simulink model "mcecu_uds_on_fusion"  (Simulink 9.2)
settings: Solver=VariableStepAuto  StartTime=0.0  StopTime=10  RelTol=1e-3
undefined symbols (not defined in the file or in its folder): canChannel
libraries: canlib x3, canmsglib x3
settings Model: Creator=cordunoalbarran  LastModifiedBy=cordunoalbarran
settings DataIOCC: LimitDataPoints=off  SaveFormat=Dataset  SignalLoggingSaveFormat=Dataset
settings OptimizationCC: DefaultParameterBehavior=Inlined  EnhancedBackFolding=on  PassReuseOutputArgsThreshold=0  LifeSpan=auto  OptimizeBlockOrder=speed  DifferentSizesBufferReuse=on  OptimizationCustomize=off
settings DebuggingCC: UnderspecifiedInitializationDetection=Simplified  MergeDetectMultiDrivingBlocksExec=error  ParameterTunabilityLossMsg=error  FcnCallInpInsideContextMsg=error  StateNameClashWarn=none  SFUnexpectedBacktrackingDiag=error  SFNoUnconditionalDefaultTransitionDiag=error  SFExecutionAtInitializationDiag=warning
settings HardwareCC: ProdBitPerPointer=64  ProdBitPerSizeT=64  ProdBitPerPtrDiffT=64  ProdLargestAtomicFloat=Float  ProdIntDivRoundTo=Zero  ProdEndianess=LittleEndian  ProdWordSize=64  ProdHWDeviceType=Intel->x86-64 (Windows64)
settings ModelReferenceCC: PropagateSignalLabelsOutOfModel=on
settings SFSimCC: SimUseLocalCustomCode=on  MATLABDynamicMemAlloc=off
settings RTWCC: GenerateReport=on  RTWUseLocalCustomCode=on  LaunchReport=on
settings CodeAppCC: ForceParamTrailComments=on  OperatorAnnotations=on  StateflowObjectComments=off
settings GRTTargetCC: TargetLangStandard=C99 (ISO)  GeneratePreprocessorConditionals=Use local settings  CombineOutputUpdateFcns=on  GRTInterface=off
settings ConfigComp: CovMetricSettings=dwe  CovHtmlReporting=off  CovSaveCumulativeToWorkspaceVar=off  CovSaveSingleToWorkspaceVar=off  CovExternalEMLEnable=on

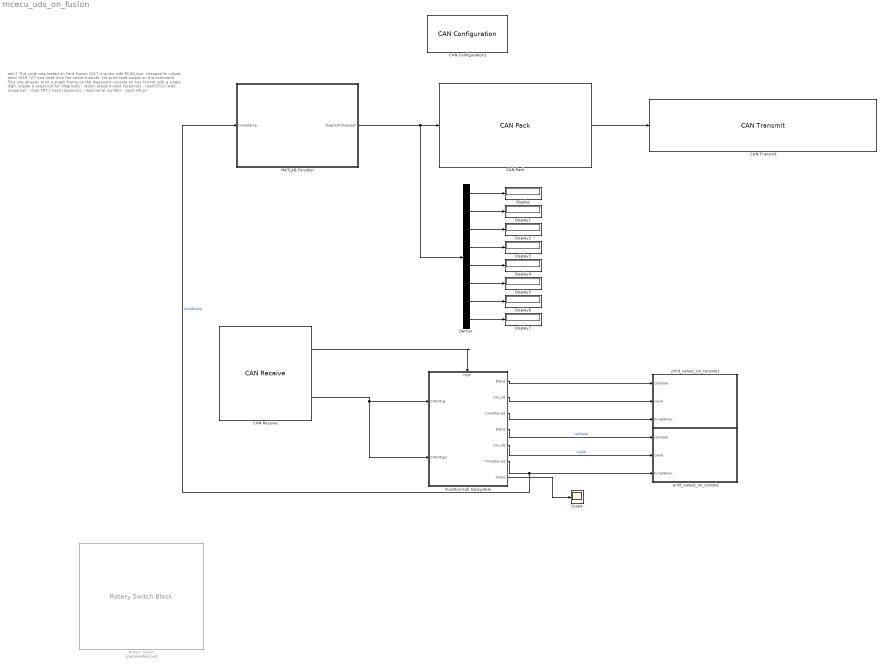
== system mcecu_uds_on_fusion ==
  note: abr/7 This code was tested on Ford Fusion 2017
      | it works with PCAN tool.
      | changed to virtual.
      | send 1959-7A7 and read it on the same channel.
      |
      | 1st print read output on the command. This one already print a single frame on the diagnostic console on hex format with a single digit.
      |
      | create a sequence for diagnostic
      |
      | - tester present (wait response)
      | - read DTCs (wait response)
      | - clear DTCs (wait response)
      | - read serial number
      | - read SW pn
      |
      | -
  CAN Configuration1 : canlib/CAN Configuration  BlockHandle=4.0002  DeviceMenu=MathWorks Virtual 1 (Channel 1)  Device=MathWorks Virtual 1 (Channel 1)  ObjConstructor=canChannel('MathWorks', 'Virtual 1', 1)  BusSpeed=500000  EnableBitParameters=off  AckMode=Normal
      settings: SourceProductName=Vehicle Network Toolbox  SourceProductBaseCode=VN
  CAN Pack : canmsglib/CAN Pack  CANdbFile=C:\Users\cordunoalbarran\Documents\GUv0 Design Docs\CAN\ccan_diagnostic.dbc  MsgList=D_RQ_FUSION_CC  MsgName=D_RQ_FUSION_CC  MsgIDType=Standard (11-bit identifier)  MsgIdentifier=1959  MsgLength=8  SignalInfo=D_RQ_FUSION_CC$56$64$2$2$1$0$1$0$-Inf$Inf$#  NSignals=1  StartBits=str2num('[int32(56)]')  SignalSizes=str2num('[int32(64)]')  ByteOrders=str2num('[int32(2)]')  DataTypes=str2num('[int32(2)]')  MultiplexTypes=str2num('[int32(1)]')  MultiplexValues=str2num('[double(0)]')  Factors=str2num('[double(1)]')  Offsets=str2num('[double(0)]')  Minimums=str2num('[double(-Inf)]')  Maximums=str2num('[double(Inf)]')  Remote=off  ApplyMinMax=off  BusOutput=off
      settings: SourceProductName=Simulink Real-Time  SourceProductBaseCode=XP  DataFormat=raw data
  CAN Receive : canlib/CAN Receive  BlockHandle=6.0002  DeviceMenu=MathWorks Virtual 1 (Channel 1)  Device=MathWorks Virtual 1 (Channel 1)  ObjConstructor=canChannel('MathWorks', 'Virtual 1', 1)  EnableStandardIDsFilter=off  StandardIDs=0  EnableExtendedIDsFilter=off  ExtendedIDs=0  SampleTime=0.001  MsgsPerTimestep=all  StdIDsCombo=Allow all  ExtIDsCombo=Allow all  InternalFilterUpdateStatus=on  BusOutput=off
      settings: SourceProductName=Vehicle Network Toolbox  SourceProductBaseCode=VN
  CAN Transmit : canlib/CAN Transmit  BlockHandle=7.0002  DeviceMenu=MathWorks Virtual 1 (Channel 1)  Device=MathWorks Virtual 1 (Channel 1)  ObjConstructor=canChannel('MathWorks', 'Virtual 1', 1)  EnablePeriodicTransmit=on  MessagePeriod=1
      settings: SourceProductName=Vehicle Network Toolbox  SourceProductBaseCode=VN
  Demux : Demux  Outputs=8
  Display{,1..7} (8 alike) : Display
  Function-Call Subsystem : Subsystem  TreatAsAtomicUnit=on
  MATLAB Function : MATLAB Function  TreatAsAtomicUnit=on
  Rotary Switch : RotarySwitchBlock  Commented=on  WebBlockId=5  Values=DataTag0
  Scope : Scope
  print_values_on_console : MATLAB Function  TreatAsAtomicUnit=on
  print_values_on_console1 : MATLAB Function  TreatAsAtomicUnit=on
  wires:
  CAN Receive/2 -> Function-Call Subsystem/2(CAN Msg1), Function-Call Subsystem/1(CAN Msg)
  CAN Receive/1 -> Function-Call Subsystem/Trigger
  MATLAB Function/1(diagnosticRequest) -> Demux/1, CAN Pack/1
  Demux/1 -> Display/1
  Demux/2 -> Display1/1
  Demux/3 -> Display2/1
  Demux/4 -> Display3/1
  Demux/5 -> Display4/1
  Demux/6 -> Display5/1
  Demux/7 -> Display6/1
  Demux/8 -> Display7/1
  Function-Call Subsystem/1(Data1) -> print_values_on_console1/1(canData)
  Function-Call Subsystem/2(can_id1) -> print_values_on_console1/2(canId)
  Function-Call Subsystem/4(Data2) -> print_values_on_console/1(canData)  "canData"
  Function-Call Subsystem/5(can_id2) -> print_values_on_console/2(canId)  "CanId"
  Function-Call Subsystem/6(Timestamp2) -> print_values_on_console/3(timeStamp), MATLAB Function/1(timeStamp)  "timeStamp"
  Function-Call Subsystem/3(timeStamp1) -> print_values_on_console1/3(timeStamp)
  CAN Pack/1 -> CAN Transmit/1
  Function-Call Subsystem/7(status) -> Scope/1

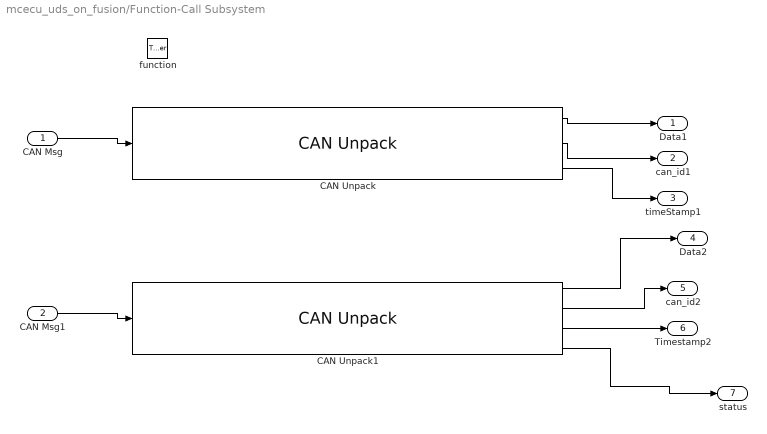
== system mcecu_uds_on_fusion/Function-Call Subsystem ==
  CAN Msg : Inport
  CAN Msg1 : Inport  Port=2
  function : TriggerPort  TriggerType=function-call  VariantControl=Variant
  CAN Unpack : canmsglib/CAN Unpack  CANdbFile=C:\Users\cordunoalbarran\Documents\GUv0 Design Docs\CAN\ccan_diagnostic.dbc  MsgList=D_RS_FUSION_CC  MsgName=D_RS_FUSION_CC  MsgIDType=Standard (11-bit identifier)  MsgIdentifier=1967  MsgLength=8  SignalInfo=D_RS_FUSION_CC$56$64$2$2$1$0$1$0$-Inf$Inf$#  NSignals=1  IDPort=on  TimestampPort=on  ErrorPort=off  RemotePort=off  LengthPort=off  StatusPort=off  StartBits=str2num('[int32(56)]')  SignalSizes=str2num('[int32(64)]')  ByteOrders=str2num('[int32(2)]')  DataTypes=str2num('[int32(2)]')  MultiplexTypes=str2num('[int32(1)]')  MultiplexValues=str2num('[double(0)]')  Factors=str2num('[double(1)]')  Offsets=str2num('[double(0)]')  Minimums=str2num('[double(-Inf)]')  Maximums=str2num('[double(Inf)]')  ApplyMinMax=off
      settings: SourceProductName=Simulink Real-Time  SourceProductBaseCode=XP  DataFormat=raw data
  CAN Unpack1 : canmsglib/CAN Unpack  CANdbFile=C:\Users\cordunoalbarran\Documents\GUv0 Design Docs\CAN\ccan_diagnostic.dbc  MsgList=D_RQ_FUSION_CC  MsgName=D_RQ_FUSION_CC  MsgIDType=Standard (11-bit identifier)  MsgIdentifier=1959  MsgLength=8  SignalInfo=D_RS_FUSION_CC$56$64$2$2$1$0$1$0$-Inf$Inf$#  NSignals=1  IDPort=on  TimestampPort=on  ErrorPort=off  RemotePort=off  LengthPort=off  StatusPort=on  StartBits=str2num('[int32(56)]')  SignalSizes=str2num('[int32(64)]')  ByteOrders=str2num('[int32(2)]')  DataTypes=str2num('[int32(2)]')  MultiplexTypes=str2num('[int32(1)]')  MultiplexValues=str2num('[double(0)]')  Factors=str2num('[double(1)]')  Offsets=str2num('[double(0)]')  Minimums=str2num('[double(-Inf)]')  Maximums=str2num('[double(Inf)]')  ApplyMinMax=off
      settings: SourceProductName=Simulink Real-Time  SourceProductBaseCode=XP  DataFormat=raw data
  Data1 : Outport
  can_id1 : Outport  Port=2  VectorParamsAs1DForOutWhenUnconnected=on
  timeStamp1 : Outport  Port=3  VectorParamsAs1DForOutWhenUnconnected=on
  Data2 : Outport  Port=4
  can_id2 : Outport  Port=5  VectorParamsAs1DForOutWhenUnconnected=on
  Timestamp2 : Outport  Port=6
  status : Outport  Port=7
  wires:
  CAN Msg/1 -> CAN Unpack/1
  CAN Unpack/1 -> Data1/1
  CAN Unpack/2 -> can_id1/1
  CAN Unpack1/1 -> Data2/1
  CAN Msg1/1 -> CAN Unpack1/1
  CAN Unpack1/2 -> can_id2/1
  CAN Unpack1/3 -> Timestamp2/1
  CAN Unpack/3 -> timeStamp1/1
  CAN Unpack1/4 -> status/1

== matlab function print_values_on_console1 ==
  data: canData input double; canId input double; timeStamp input double
function display_7AF(canData, canId, timeStamp)

mcecu_uds_on_fusion.displayCanMsgOnConsole( ...
    canData, canId, timeStamp);

% fprintf('%.5f', timeStamp);
% fprintf(' %X', canId);  %; with colom is printed on the diagnostic console
% for i = 1 : numel(canData)
%     strData = canData(i);
%     if i == numel(canData)
%         fprintf(' %X\n', strData);
%     else
%         fprintf(' %X', strData);
%     end
% end    

% %CAN diagnostic data length
% dataLengh = 8;
% 
% fprintf('%X', canId);  %; with colom is printed on the diagnostic console
% for i = 1:numel(canData)
%     strData = canData(i);
%     if i == dataLengh
%         fprintf(' %X\n', strData);
%     else
%         fprintf(' %X', strData);
%     end
% end

== matlab function print_values_on_console ==
  data: canData input double; canId input double; timeStamp input double
function display_7A7(canData, canId, timeStamp)

mcecu_uds_on_fusion.displayCanMsgOnConsole( ...
    canData, canId, timeStamp);

== matlab function MATLAB Function ==
  data: diagnosticRequest output uint8; timeStamp input double
function diagnosticRequest = createDiagnosticVectors(timeStamp)

diagnosticRequest= mcecu_uds_on_fusion.createDiagnosticVectors(timeStamp); %this one compile and send a vector
